simulink model "MotordcPID"  (R2013a)
settings: Solver=ode45  StartTime=0.0  StopTime=100  RelTol=1e-3
values from neighbouring files (symbols this model uses):
  Den1 = [(La1*Jm1) ((Ra1*Jm1)+(Bm1*La1)) ((Ra1*Bm1)+(ki1*kv1))]    [PIDproy3.m]
  Num1 = [ki1]    [PIDproy3.m]
libraries: simulink_need_slupdate x1
settings Model: Creator=user  LastModifiedBy=user

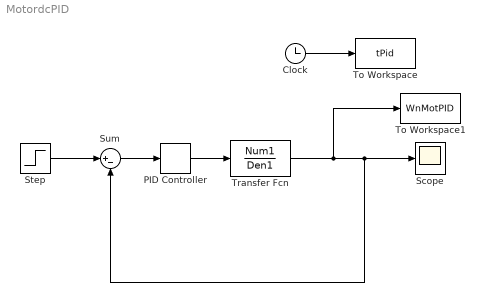
== system MotordcPID ==
  Clock : Clock
  PID Controller : simulink_need_slupdate/PID Controller  P=0.5  I=0  D=0
  Scope : Scope
  Step : Step  Time=0  After=6  SampleTime=0
  Sum : Sum  Inputs=|+-
  To Workspace : ToWorkspace  VariableName=tPid  SampleTime=-1
  To Workspace1 : ToWorkspace  VariableName=WnMotPID
  Transfer Fcn : TransferFcn  Numerator=Num1  Denominator=Den1
  wires:
  Clock/1 -> To Workspace/1
  Step/1 -> Sum/1
  Transfer Fcn/1 -> To Workspace1/1, Sum/2, Scope/1
  Sum/1 -> PID Controller/1
  PID Controller/1 -> Transfer Fcn/1
